simulink model "LimitCycle_Simulation"  (R2022b)
settings: Solver=FixedStepAuto  StartTime=0.0  StopTime=10.0  FixedStep=0.005  RelTol=1e-6
settings Model: Creator=arkad  LastModifiedBy=arkad

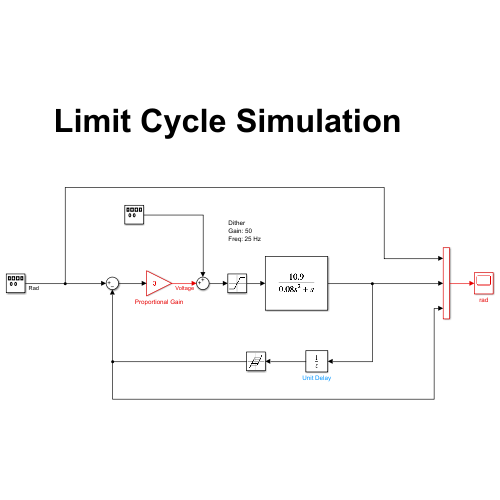
[thumbnail: Simulink's stored preview of the top-level diagram]
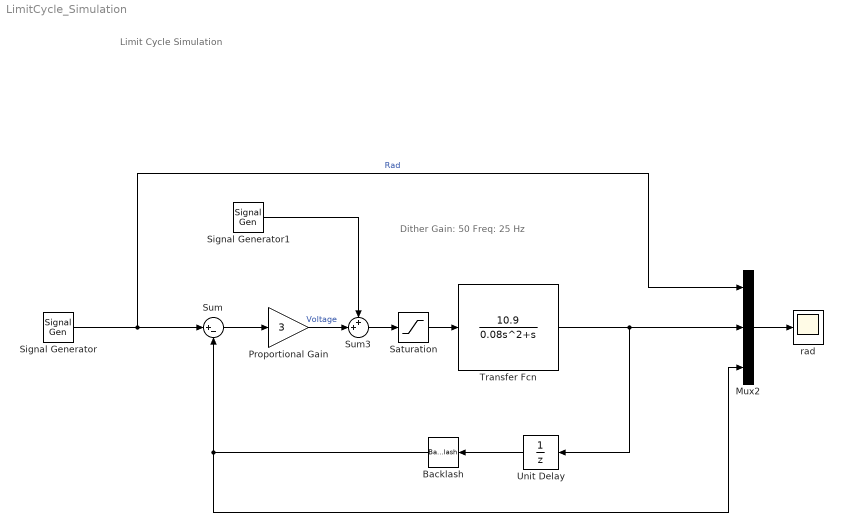
== system LimitCycle_Simulation ==
  note: Limit Cycle Simulation
  note: Dither
      | Gain: 50
      | Freq: 25 Hz
  Backlash : Backlash  BacklashWidth=0.35
  Mux2 : Mux  Inputs=3
  Proportional Gain : Gain  Gain=3
  Saturation : Saturate  UpperLimit=12  LowerLimit=-12
  Signal Generator : SignalGenerator  WaveForm=square  Frequency=0.1
  Signal Generator1 : SignalGenerator  Amplitude=15  Frequency=25
  Sum : Sum  Inputs=|+-
  Sum3 : Sum  Inputs=++|
  Transfer Fcn : TransferFcn  Numerator=[10.9]  Denominator=[0.08 1 0]
  Unit Delay : UnitDelay  SampleTime=-1  HasFrameUpgradeWarning=on
  rad : Scope
  wires:
  Signal Generator/1 -> Mux2/1, Sum/1  "Rad"
  Sum3/1 -> Saturation/1
  Signal Generator1/1 -> Sum3/1
  Sum/1 -> Proportional Gain/1
  Proportional Gain/1 -> Sum3/2  "Voltage"
  Transfer Fcn/1 -> Unit Delay/1, Mux2/2
  Mux2/1 -> rad/1
  Saturation/1 -> Transfer Fcn/1
  Unit Delay/1 -> Backlash/1
  Backlash/1 -> Mux2/3, Sum/2
